simulink model "inner_APPC_thrust_d"  (R2016a)
settings: Solver=VariableStepAuto  StartTime=0.0  StopTime=50  RelTol=1e-3
settings Model: Creator=Daniel  LastModifiedBy=mgreiff
settings DataIOCC: LimitDataPoints=on
settings DebuggingCC: AllowSymbolicDim=off
settings ModelReferenceCC: PropagateSignalLabelsOutOfModel=off
settings GRTTargetCC: GeneratePreprocessorConditionals=Use local settings

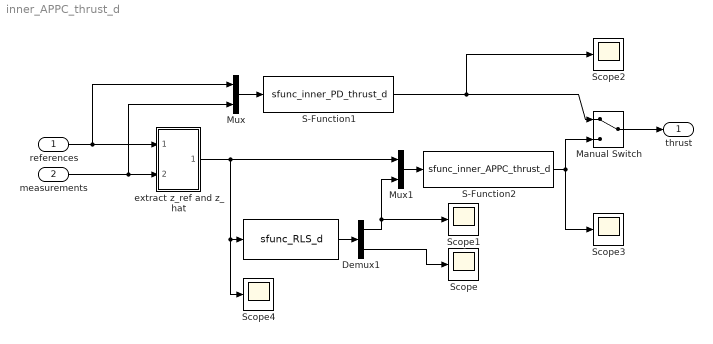
== system inner_APPC_thrust_d ==
  references : Inport  PortDimensions=12
  measurements : Inport  Port=2  PortDimensions=12
  "   " : S-Function  FunctionName=sfunc_RLS_d  Parameters=RLSparam  SFunctionDeploymentMode=off  EnableBusSupport=off
  Demux1 : Demux  Outputs=[4,1]
  Manual Switch : ManualSwitch
  Mux : Mux  Inputs=2
  Mux1 : Mux  Inputs=2
  S-Function1 : S-Function  FunctionName=sfunc_inner_PD_thrust_d  Parameters=PD_thrust_param  SFunctionDeploymentMode=off  EnableBusSupport=off
  S-Function2 : S-Function  FunctionName=sfunc_inner_APPC_thrust_d  SFunctionDeploymentMode=off  EnableBusSupport=off
  Scope{,1..4} (5 alike) : Scope
  extract z_ref and z_hat : Subsystem
  thrust : Outport
  wires:
  Mux/1 -> S-Function1/1
  S-Function1/1 -> Manual Switch/1, Scope2/1
  "   "/1 -> Demux1/1
  Mux1/1 -> S-Function2/1
  Demux1/1 -> Mux1/2, Scope1/1
  Demux1/2 -> Scope/1
  S-Function2/1 -> Manual Switch/2, Scope3/1
  references/1 -> extract z_ref and z_hat/1(In1), Mux/1
  extract z_ref and z_hat/1(Out1) -> Mux1/1, Scope4/1, "   "/1
  Manual Switch/1 -> thrust/1
  measurements/1 -> Mux/2, extract z_ref and z_hat/2(In2)

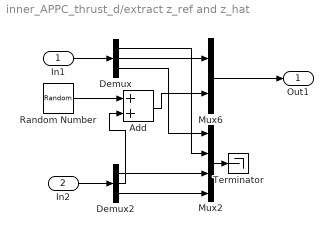
== system inner_APPC_thrust_d/extract z_ref and z_hat ==
  In1 : Inport
  In2 : Inport  Port=2
  Add : Sum
  Demux : Demux  Outputs=[2,1,9]
  Demux2 : Demux  Outputs=[2,1,9]
  Mux2 : Mux
  Mux6 : Mux  Inputs=2
  Random Number : RandomNumber  Variance=0.1  SampleTime=0.002
  Terminator : Terminator
  Out1 : Outport
  wires:
  Mux6/1 -> Out1/1
  In1/1 -> Demux/1
  Demux/3 -> Mux2/1
  Demux/1 -> Mux2/2
  Demux2/3 -> Mux2/4
  Demux/2 -> Mux6/1
  Demux2/1 -> Mux2/3
  In2/1 -> Demux2/1
  Mux2/1 -> Terminator/1
  Random Number/1 -> Add/1
  Add/1 -> Mux6/2
  Demux2/2 -> Add/2
